simulink model "HANcoder_E407_GTSync_v6"  (R2018b)
settings: Solver=FixedStepDiscrete  StartTime=0.0  StopTime=1  FixedStep=0.01  RelTol=1e-3
PreLoadFcn:
  | librarySetup
  | eval([bdroot,'_startup']) %Calling [modelName]_startup.m
values from neighbouring files (symbols this model uses):
  basic_cycle_duration = TM_Reset_Board + COMP_duration    (= 212)    [HANcoder_E407_GTSync_v6_startup.m]
  comm_delay_estimation1 = round(comm_delay_measured1*hardware_granularity/frequency_IRQ)    [HANcoder_E407_GTSync_v6_startup.m]
  comm_delay_estimation2 = round(comm_delay_measured2*hardware_granularity/frequency_IRQ)    [HANcoder_E407_GTSync_v6_startup.m]
  COMM_Period = 40    [HANcoder_E407_GTSync_v6_startup.m]
  COMM_Phase1 = 5    [HANcoder_E407_GTSync_v6_startup.m]
  COMM_Phase2 = 8    [HANcoder_E407_GTSync_v6_startup.m]
  frequency_IRQ = 100    [HANcoder_E407_GTSync_v6_startup.m]
  HANtuneOverride = Simulink.Parameter    [HANcoder_E407_GTSync_v6_startup.m]
  idle_time_init = basic_cycle_duration*matrix_rows    (= 424)    [HANcoder_E407_GTSync_v6_startup.m]
  LA_COMM_Err = 1    [HANcoder_E407_GTSync_v6_startup.m]
  LA_MEX_Flag = 0    [HANcoder_E407_GTSync_v6_startup.m]
  LA_Task_Act = 1    [HANcoder_E407_GTSync_v6_startup.m]
  LED_ticks_toggle = 10000    [HANcoder_E407_GTSync_v6_startup.m]
  Master_Role = 1    [HANcoder_E407_GTSync_v6_startup.m]
  matrix_rows = 2    [HANcoder_E407_GTSync_v6_startup.m]
  max_num_msgs_CAN1 = 2^Tx_bit_number-1    (= 7)    [HANcoder_E407_GTSync_v6_startup.m]
  max_num_msgs_CAN2 = max_num_msgs_CAN1    (= 7)    [HANcoder_E407_GTSync_v6_startup.m]
  Slave_Role = 2    [HANcoder_E407_GTSync_v6_startup.m]
  Sync_ID = 1    [HANcoder_E407_GTSync_v6_startup.m]
  TM_Check_Sync = TM_COMM_Sync   + COMM_duration    (= 40)    [HANcoder_E407_GTSync_v6_startup.m]
  TM_Check_TOuts = TM_Count_Vote3 + COMP_duration    (= 196)    [HANcoder_E407_GTSync_v6_startup.m]
  TM_Check_Vote1 = TM_COMM_Vote1  + COMM_duration    (= 92)    [HANcoder_E407_GTSync_v6_startup.m]
  TM_Check_Vote2 = TM_COMM_Vote2  + COMM_duration    (= 140)    [HANcoder_E407_GTSync_v6_startup.m]
  TM_Check_Vote3 = TM_COMM_Vote3  + COMM_duration    (= 188)    [HANcoder_E407_GTSync_v6_startup.m]
  TM_COMM_Sync = basic_cycle_start    (= 0)    [HANcoder_E407_GTSync_v6_startup.m]
  TM_COMM_Vote1 = TM_Vote_Dec    + COMP_duration    (= 52)    [HANcoder_E407_GTSync_v6_startup.m]
  TM_COMM_Vote2 = TM_Count_Vote1 + COMP_duration    (= 100)    [HANcoder_E407_GTSync_v6_startup.m]
  TM_COMM_Vote3 = TM_Count_Vote2 + COMP_duration    (= 148)    [HANcoder_E407_GTSync_v6_startup.m]
  TM_Count_Vote1 = TM_Check_Vote1 + COMP_duration    (= 96)    [HANcoder_E407_GTSync_v6_startup.m]
  TM_Count_Vote2 = TM_Check_Vote2 + COMP_duration    (= 144)    [HANcoder_E407_GTSync_v6_startup.m]
  TM_Count_Vote3 = TM_Check_Vote3 + COMP_duration    (= 192)    [HANcoder_E407_GTSync_v6_startup.m]
  TM_Data = TM_COMM_Sync    (= 0)    [HANcoder_E407_GTSync_v6_startup.m]
  TM_New_Master = TM_Check_TOuts + COMP_duration    (= 200)    [HANcoder_E407_GTSync_v6_startup.m]
  TM_Reset_Board = TM_Reset_Var   + COMP_duration    (= 208)    [HANcoder_E407_GTSync_v6_startup.m]
  TM_Reset_Var = TM_New_Master  + COMP_duration    (= 204)    [HANcoder_E407_GTSync_v6_startup.m]
  TM_Type = COMM    (= 0)    [HANcoder_E407_GTSync_v6_startup.m]
  TM_Update_LT = TM_Check_Sync  + COMP_duration    (= 44)    [HANcoder_E407_GTSync_v6_startup.m]
  TM_Vote_Dec = TM_Update_LT   + COMP_duration    (= 48)    [HANcoder_E407_GTSync_v6_startup.m]
  Vote1_ID = 11    [HANcoder_E407_GTSync_v6_startup.m]
  Vote2_ID = 12    [HANcoder_E407_GTSync_v6_startup.m]
  Vote3_ID = 13    [HANcoder_E407_GTSync_v6_startup.m]
undefined symbols (not defined in the file or in its folder): A0, A1, A2, A3, CON2
libraries: hdlsllib x75, HANcoder_STM32_Target x25, simulink x3, simulink_extras x1
(part 3 of 8)

== system HANcoder_E407_GTSync_v6/HANcoder STM32 Target - E407-STM32 algorithm/Global Ticks Increment/CAN Management/Initialization/RoleID and Global Time init ==
  note: Sync msg received!
  note: Reset variables
  note: Finish Initialization
  note: Role_ID Initialization
  Timeout Initialization : Inport
  Reference message received : Inport  Port=2
  Enable : EnablePort
  Constant : Constant  Priority=4  Value=Master_Role
  Constant1 : Constant  Priority=3  Value=Slave_Role
  Data Store Read : DataStoreRead  Priority=5  DataStoreName=Role_ID
  Data Store Write : DataStoreWrite  Priority=8  DataStoreName=Role_ID
  Data Store Write2 : DataStoreWrite  Priority=18  DataStoreName=Delay_Counter
  Data Store Write3 : DataStoreWrite  Priority=12  DataStoreName=New_Msg_Ready_CAN1
  Data Store Write4 : DataStoreWrite  Priority=16  DataStoreName=Initialization_Timeout
  Data Store Write5 : DataStoreWrite  Priority=14  DataStoreName=New_Msg_Ready_CAN2
  Global Time Initialization Master : Subsystem  Priority=2
  Global Time Initialization Slave : Subsystem  Priority=1
  RESET : Constant  Priority=15  Value=0  OutDataTypeStr=boolean
  RESET1 : Constant  Priority=17  Value=0  OutDataTypeStr=double
  RESET2 : Constant  Priority=11  Value=0  OutDataTypeStr=boolean
  RESET3 : Constant  Priority=13  Value=0  OutDataTypeStr=boolean
  SET : Constant  Priority=19
  Switch1 : Switch  Priority=6  Criteria=u2 > Threshold
  Switch2 : Switch  Priority=7  Criteria=u2 > Threshold
  Finish Initialization : Outport  OutputWhenDisabled=reset  InitialOutput=0
  wires:
  Switch1/1 -> Switch2/3
  Reference message received/1 -> Global Time Initialization Slave/Enable, Switch2/2
  Data Store Read/1 -> Switch1/3
  SET/1 -> Finish Initialization/1
  Constant/1 -> Switch1/1
  Constant1/1 -> Switch2/1
  Switch2/1 -> Data Store Write/1
  RESET/1 -> Data Store Write4/1
  Timeout Initialization/1 -> Switch1/2, Global Time Initialization Master/Enable
  RESET1/1 -> Data Store Write2/1
  RESET2/1 -> Data Store Write3/1
  RESET3/1 -> Data Store Write5/1

== system HANcoder_E407_GTSync_v6/HANcoder STM32 Target - E407-STM32 algorithm/Global Ticks Increment/CAN Management/LT_Update Desync_Positive/Local Time Update with Positive Desync ==
  note: Positive Desync with respect to the master
      | If the desync is positive, we have to update the
      | Local Time to be "in the future". This is problematic
      | because we do not want the schedule to go ahead
      | of time and forget to do any task. That is why we
      | correct the desync in small steps.
  note: End condition
  note: Desync counter
      | reduction
  note: Local Time Update
  note: Current Local Time correction
  Ticks until next COMP : Inport
  Cast : DataTypeConversion  Priority=13  OutDataTypeStr=uint16
  Constant : Constant  Value=0
  Data Store Read : DataStoreRead  DataStoreName=Local_Ticks
  Data Store Read2 : DataStoreRead  DataStoreName=Desync_Ticks
  Data Store Write : DataStoreWrite  DataStoreName=Desync_Positive
  Data Store Write1 : DataStoreWrite  Priority=14  DataStoreName=Local_Ticks  DataStoreElements=Local_Ticks
  Data Store Write2 : DataStoreWrite  DataStoreName=Desync_Ticks
  Equal : RelationalOperator  Operator=<=  OutDataTypeStr=boolean  RndMeth=Simplest
  GreaterThan : RelationalOperator  Operator=<=  OutDataTypeStr=boolean  RndMeth=Simplest
  Minus : Sum  Priority=12
  Minus1 : Sum  Inputs=+-
  NOT : Logic  Operator=NOT  IconShape=distinctive  AllPortsSameDT=off  OutDataTypeStr=boolean
  Switch : Switch  Criteria=u2 > Threshold
  wires:
  Ticks until next COMP/1 -> Switch/1, GreaterThan/1
  Data Store Read/1 -> Minus/1
  Cast/1 -> Data Store Write1/1
  Minus/1 -> Cast/1
  Data Store Read2/1 -> Switch/3, GreaterThan/2, Minus1/2
  Minus1/1 -> Equal/1, Data Store Write2/1
  Constant/1 -> Equal/2
  Equal/1 -> NOT/1
  NOT/1 -> Data Store Write/1
  GreaterThan/1 -> Switch/2
  Switch/1 -> Minus1/1, Minus/2

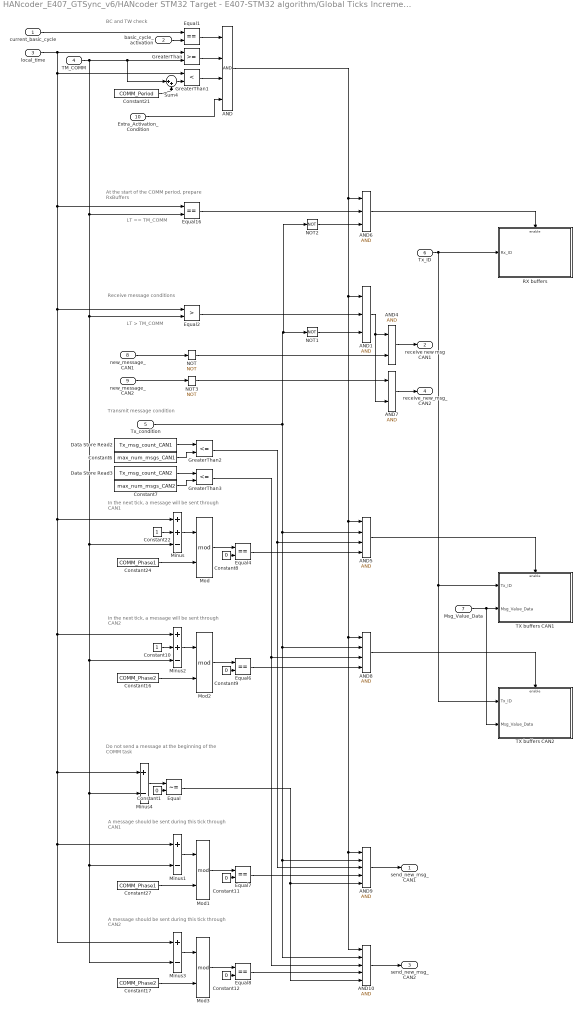
== system HANcoder_E407_GTSync_v6/HANcoder STM32 Target - E407-STM32 algorithm/Global Ticks Increment/CAN Management/Matrix Cycle Manager/COMM Task - Sync BC0 ==
  note: Do not send a message at the
      | beginning of the COMM task
  note: LT > TM_COMM
  note: At the start of the COMM
      | period, prepare RxBuffers
  note: In the next tick, a message will be
      | sent through CAN1
  note: BC and TW check
  note: Receive message conditions
  note: A message should be sent during
      | this tick through CAN1
  note: In the next tick, a message will be
      | sent through CAN2
  note: Transmit message condition
  note: A message should be sent during
      | this tick through CAN2
  note: LT == TM_COMM
  current_basic_cycle : Inport
  basic_cycle_activation : Inport  Port=2
  local_time : Inport  Port=3
  TM_COMM : Inport  Port=4
  Tx_condition : Inport  Port=5
  Tx_ID : Inport  Port=6
  Msg_Value_Data : Inport  Port=7
  new_message_CAN1 : Inport  Port=8
  new_message_CAN2 : Inport  Port=9
  Extra_Activation_Condition : Inport  Port=10
  AND : Logic  Inputs=4  IconShape=distinctive  AllPortsSameDT=off  OutDataTypeStr=boolean
  AND1 : Logic  Inputs=3  IconShape=distinctive  AllPortsSameDT=off  OutDataTypeStr=boolean
  AND10 : Logic  Inputs=5  IconShape=distinctive  AllPortsSameDT=off  OutDataTypeStr=boolean
  AND4 : Logic  IconShape=distinctive  AllPortsSameDT=off  OutDataTypeStr=boolean
  AND5 : Logic  Inputs=4  IconShape=distinctive  AllPortsSameDT=off  OutDataTypeStr=boolean
  AND6 : Logic  Inputs=3  IconShape=distinctive  AllPortsSameDT=off  OutDataTypeStr=boolean
  AND7 : Logic  IconShape=distinctive  AllPortsSameDT=off  OutDataTypeStr=boolean
  AND8 : Logic  Inputs=4  IconShape=distinctive  AllPortsSameDT=off  OutDataTypeStr=boolean
  AND9 : Logic  Inputs=5  IconShape=distinctive  AllPortsSameDT=off  OutDataTypeStr=boolean
  Constant{1,8..9,11..12} (5 alike) : Constant  Value=0
  Constant10 : Constant
  Constant16 : Constant  Value=COMM_Phase2
  Constant17 : Constant  Value=COMM_Phase2
  Constant21 : Constant  Value=COMM_Period
  Constant22 : Constant
  Constant24 : Constant  Value=COMM_Phase1
  Constant27 : Constant  Value=COMM_Phase1
  Constant6 : Constant  Value=max_num_msgs_CAN1
  Constant7 : Constant  Value=max_num_msgs_CAN2
  Data Store Read2 : DataStoreRead  DataStoreName=Tx_msg_count_CAN1
  Data Store Read3 : DataStoreRead  DataStoreName=Tx_msg_count_CAN2
  Equal : RelationalOperator  Operator=~=  OutDataTypeStr=boolean  RndMeth=Simplest
  Equal{1,4,6..8,16} (6 alike) : RelationalOperator  Operator===  OutDataTypeStr=boolean  RndMeth=Simplest
  Equal2 : RelationalOperator  Operator=>  OutDataTypeStr=boolean  RndMeth=Simplest
  GreaterThan : RelationalOperator  OutDataTypeStr=boolean  RndMeth=Simplest
  GreaterThan1 : RelationalOperator  Operator=<  OutDataTypeStr=boolean  RndMeth=Simplest
  GreaterThan2 : RelationalOperator  Operator=<=  OutDataTypeStr=boolean  RndMeth=Simplest
  GreaterThan3 : RelationalOperator  Operator=<=  OutDataTypeStr=boolean  RndMeth=Simplest
  Minus : Sum  Inputs=++-
  Minus1 : Sum  Inputs=+-
  Minus2 : Sum  Inputs=++-
  Minus3 : Sum  Inputs=+-
  Minus4 : Sum  Inputs=+-
  Mod{,1..3} (4 alike) : Math  Operator=mod  SaturateOnIntegerOverflow=on
  NOT{,1..3} (4 alike) : Logic  Operator=NOT  IconShape=distinctive  AllPortsSameDT=off  OutDataTypeStr=boolean
  RX buffers : Subsystem  Priority=20
  Sum4 : Sum  Inputs=|++
  TX buffers CAN1 : Subsystem  Priority=20
  TX buffers CAN2 : Subsystem  Priority=20
  send_new_msg_CAN1 : Outport
  receive new msg CAN1 : Outport  Port=2
  send_new_msg_CAN2 : Outport  Port=3
  receive_new_msg_CAN2 : Outport  Port=4
  wires:
  basic_cycle_activation/1 -> Equal1/2
  new_message_CAN1/1 -> NOT/1
  current_basic_cycle/1 -> Equal1/1
  Constant21/1 -> Sum4/2
  Sum4/1 -> GreaterThan1/2
  Equal1/1 -> AND/1
  GreaterThan/1 -> AND/2
  GreaterThan1/1 -> AND/3
  AND5/1 -> TX buffers CAN1/Enable
  Constant22/1 -> Minus/2
  Minus/1 -> Mod/1
  Constant24/1 -> Mod/2
  Constant27/1 -> Mod1/2
  Minus1/1 -> Mod1/1
  Equal16/1 -> AND6/2
  AND6/1 -> RX buffers/Enable
  NOT3/1 -> AND7/1
  new_message_CAN2/1 -> NOT3/1
  Equal2/1 -> AND1/2
  Tx_condition/1 -> NOT2/1, NOT1/1, AND10/2, AND9/2, AND8/2, AND5/2
  AND1/1 -> AND4/1, AND7/2
  NOT/1 -> AND4/2
  AND4/1 -> receive new msg CAN1/1
  AND7/1 -> receive_new_msg_CAN2/1
  Constant16/1 -> Mod2/2
  Minus2/1 -> Mod2/1
  Constant10/1 -> Minus2/2
  AND8/1 -> TX buffers CAN2/Enable
  AND9/1 -> send_new_msg_CAN1/1
  AND10/1 -> send_new_msg_CAN2/1
  AND/1 -> AND8/1, AND9/1, AND10/1, AND5/1, AND1/1, AND6/1
  TM_COMM/1 -> Minus/3, Minus2/3, Minus4/2, Minus3/2, Minus1/2, Equal2/2, Equal16/2, Sum4/1, GreaterThan/2
  Minus3/1 -> Mod3/1
  Constant17/1 -> Mod3/2
  Data Store Read2/1 -> GreaterThan2/1
  Constant6/1 -> GreaterThan2/2
  Constant7/1 -> GreaterThan3/2
  Data Store Read3/1 -> GreaterThan3/1
  GreaterThan2/1 -> AND9/3, AND5/3
  GreaterThan3/1 -> AND10/3, AND8/3
  Equal4/1 -> AND5/4
  Mod/1 -> Equal4/1
  Constant8/1 -> Equal4/2
  Constant9/1 -> Equal6/2
  Mod2/1 -> Equal6/1
  Constant11/1 -> Equal7/2
  Constant12/1 -> Equal8/2
  Mod3/1 -> Equal8/1
  Mod1/1 -> Equal7/1
  Equal6/1 -> AND8/4
  Equal7/1 -> AND9/4
  Equal8/1 -> AND10/4
  Tx_ID/1 -> RX buffers/1(Rx_ID), TX buffers CAN1/1(Tx_ID), TX buffers CAN2/1(Tx_ID)
  NOT1/1 -> AND1/3
  Extra_Activation_Condition/1 -> AND/4
  Msg_Value_Data/1 -> TX buffers CAN2/2(Msg_Value_Data), TX buffers CAN1/2(Msg_Value_Data)
  local_time/1 -> GreaterThan1/1, Equal16/1, Equal2/1, Minus3/1, Minus1/1, Minus4/1, Minus2/1, Minus/1, GreaterThan/1
  NOT2/1 -> AND6/3
  Constant1/1 -> Equal/2
  Minus4/1 -> Equal/1
  Equal/1 -> AND10/5, AND9/5

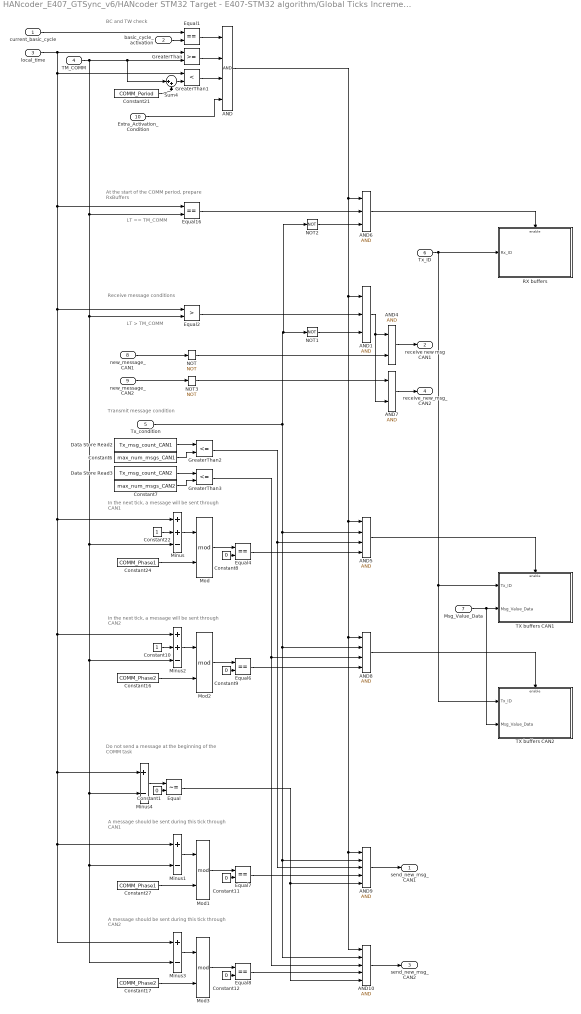
== system HANcoder_E407_GTSync_v6/HANcoder STM32 Target - E407-STM32 algorithm/Global Ticks Increment/CAN Management/Matrix Cycle Manager/COMM Task - Sync BC1 ==
  note: Do not send a message at the
      | beginning of the COMM task
  note: LT > TM_COMM
  note: At the start of the COMM
      | period, prepare RxBuffers
  note: In the next tick, a message will be
      | sent through CAN1
  note: BC and TW check
  note: Receive message conditions
  note: A message should be sent during
      | this tick through CAN1
  note: In the next tick, a message will be
      | sent through CAN2
  note: Transmit message condition
  note: A message should be sent during
      | this tick through CAN2
  note: LT == TM_COMM
  current_basic_cycle : Inport
  basic_cycle_activation : Inport  Port=2
  local_time : Inport  Port=3
  TM_COMM : Inport  Port=4
  Tx_condition : Inport  Port=5
  Tx_ID : Inport  Port=6
  Msg_Value_Data : Inport  Port=7
  new_message_CAN1 : Inport  Port=8
  new_message_CAN2 : Inport  Port=9
  Extra_Activation_Condition : Inport  Port=10
  AND : Logic  Inputs=4  IconShape=distinctive  AllPortsSameDT=off  OutDataTypeStr=boolean
  AND1 : Logic  Inputs=3  IconShape=distinctive  AllPortsSameDT=off  OutDataTypeStr=boolean
  AND10 : Logic  Inputs=5  IconShape=distinctive  AllPortsSameDT=off  OutDataTypeStr=boolean
  AND4 : Logic  IconShape=distinctive  AllPortsSameDT=off  OutDataTypeStr=boolean
  AND5 : Logic  Inputs=4  IconShape=distinctive  AllPortsSameDT=off  OutDataTypeStr=boolean
  AND6 : Logic  Inputs=3  IconShape=distinctive  AllPortsSameDT=off  OutDataTypeStr=boolean
  AND7 : Logic  IconShape=distinctive  AllPortsSameDT=off  OutDataTypeStr=boolean
  AND8 : Logic  Inputs=4  IconShape=distinctive  AllPortsSameDT=off  OutDataTypeStr=boolean
  AND9 : Logic  Inputs=5  IconShape=distinctive  AllPortsSameDT=off  OutDataTypeStr=boolean
  Constant{1,8..9,11..12} (5 alike) : Constant  Value=0
  Constant10 : Constant
  Constant16 : Constant  Value=COMM_Phase2
  Constant17 : Constant  Value=COMM_Phase2
  Constant21 : Constant  Value=COMM_Period
  Constant22 : Constant
  Constant24 : Constant  Value=COMM_Phase1
  Constant27 : Constant  Value=COMM_Phase1
  Constant6 : Constant  Value=max_num_msgs_CAN1
  Constant7 : Constant  Value=max_num_msgs_CAN2
  Data Store Read2 : DataStoreRead  DataStoreName=Tx_msg_count_CAN1
  Data Store Read3 : DataStoreRead  DataStoreName=Tx_msg_count_CAN2
  Equal : RelationalOperator  Operator=~=  OutDataTypeStr=boolean  RndMeth=Simplest
  Equal{1,4,6..8,16} (6 alike) : RelationalOperator  Operator===  OutDataTypeStr=boolean  RndMeth=Simplest
  Equal2 : RelationalOperator  Operator=>  OutDataTypeStr=boolean  RndMeth=Simplest
  GreaterThan : RelationalOperator  OutDataTypeStr=boolean  RndMeth=Simplest
  GreaterThan1 : RelationalOperator  Operator=<  OutDataTypeStr=boolean  RndMeth=Simplest
  GreaterThan2 : RelationalOperator  Operator=<=  OutDataTypeStr=boolean  RndMeth=Simplest
  GreaterThan3 : RelationalOperator  Operator=<=  OutDataTypeStr=boolean  RndMeth=Simplest
  Minus : Sum  Inputs=++-
  Minus1 : Sum  Inputs=+-
  Minus2 : Sum  Inputs=++-
  Minus3 : Sum  Inputs=+-
  Minus4 : Sum  Inputs=+-
  Mod{,1..3} (4 alike) : Math  Operator=mod  SaturateOnIntegerOverflow=on
  NOT{,1..3} (4 alike) : Logic  Operator=NOT  IconShape=distinctive  AllPortsSameDT=off  OutDataTypeStr=boolean
  RX buffers : Subsystem  Priority=20
  Sum4 : Sum  Inputs=|++
  TX buffers CAN1 : Subsystem  Priority=20
  TX buffers CAN2 : Subsystem  Priority=20
  send_new_msg_CAN1 : Outport
  receive new msg CAN1 : Outport  Port=2
  send_new_msg_CAN2 : Outport  Port=3
  receive_new_msg_CAN2 : Outport  Port=4
  wires:
  basic_cycle_activation/1 -> Equal1/2
  new_message_CAN1/1 -> NOT/1
  current_basic_cycle/1 -> Equal1/1
  Constant21/1 -> Sum4/2
  Sum4/1 -> GreaterThan1/2
  Equal1/1 -> AND/1
  GreaterThan/1 -> AND/2
  GreaterThan1/1 -> AND/3
  AND5/1 -> TX buffers CAN1/Enable
  Constant22/1 -> Minus/2
  Minus/1 -> Mod/1
  Constant24/1 -> Mod/2
  Constant27/1 -> Mod1/2
  Minus1/1 -> Mod1/1
  Equal16/1 -> AND6/2
  AND6/1 -> RX buffers/Enable
  NOT3/1 -> AND7/1
  new_message_CAN2/1 -> NOT3/1
  Equal2/1 -> AND1/2
  Tx_condition/1 -> NOT2/1, NOT1/1, AND10/2, AND9/2, AND8/2, AND5/2
  AND1/1 -> AND4/1, AND7/2
  NOT/1 -> AND4/2
  AND4/1 -> receive new msg CAN1/1
  AND7/1 -> receive_new_msg_CAN2/1
  Constant16/1 -> Mod2/2
  Minus2/1 -> Mod2/1
  Constant10/1 -> Minus2/2
  AND8/1 -> TX buffers CAN2/Enable
  AND9/1 -> send_new_msg_CAN1/1
  AND10/1 -> send_new_msg_CAN2/1
  AND/1 -> AND8/1, AND9/1, AND10/1, AND5/1, AND1/1, AND6/1
  TM_COMM/1 -> Minus/3, Minus2/3, Minus4/2, Minus3/2, Minus1/2, Equal2/2, Equal16/2, Sum4/1, GreaterThan/2
  Minus3/1 -> Mod3/1
  Constant17/1 -> Mod3/2
  Data Store Read2/1 -> GreaterThan2/1
  Constant6/1 -> GreaterThan2/2
  Constant7/1 -> GreaterThan3/2
  Data Store Read3/1 -> GreaterThan3/1
  GreaterThan2/1 -> AND9/3, AND5/3
  GreaterThan3/1 -> AND10/3, AND8/3
  Equal4/1 -> AND5/4
  Mod/1 -> Equal4/1
  Constant8/1 -> Equal4/2
  Constant9/1 -> Equal6/2
  Mod2/1 -> Equal6/1
  Constant11/1 -> Equal7/2
  Constant12/1 -> Equal8/2
  Mod3/1 -> Equal8/1
  Mod1/1 -> Equal7/1
  Equal6/1 -> AND8/4
  Equal7/1 -> AND9/4
  Equal8/1 -> AND10/4
  Tx_ID/1 -> RX buffers/1(Rx_ID), TX buffers CAN1/1(Tx_ID), TX buffers CAN2/1(Tx_ID)
  NOT1/1 -> AND1/3
  Extra_Activation_Condition/1 -> AND/4
  Msg_Value_Data/1 -> TX buffers CAN2/2(Msg_Value_Data), TX buffers CAN1/2(Msg_Value_Data)
  local_time/1 -> GreaterThan1/1, Equal16/1, Equal2/1, Minus3/1, Minus1/1, Minus4/1, Minus2/1, Minus/1, GreaterThan/1
  NOT2/1 -> AND6/3
  Constant1/1 -> Equal/2
  Minus4/1 -> Equal/1
  Equal/1 -> AND10/5, AND9/5

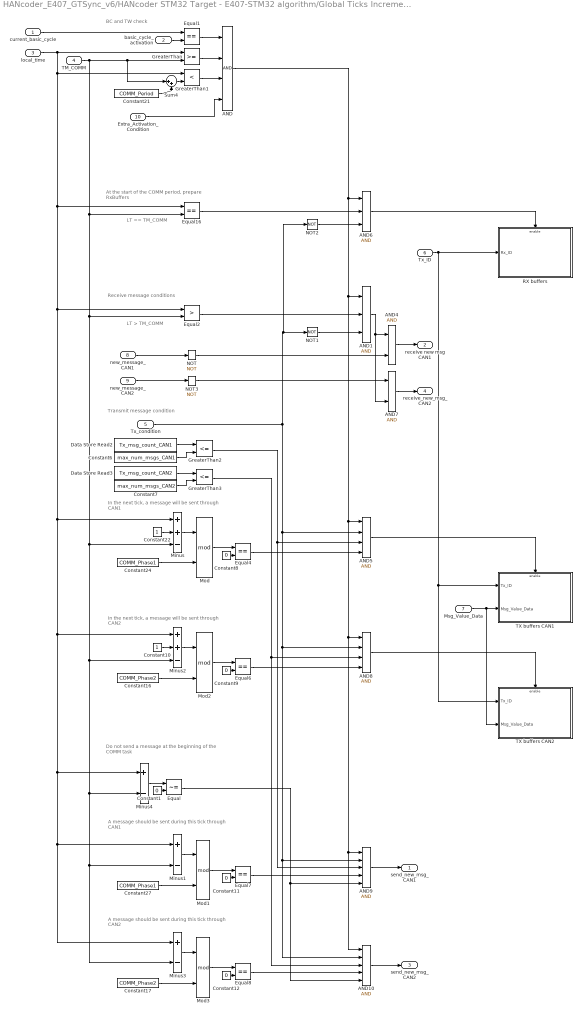
== system HANcoder_E407_GTSync_v6/HANcoder STM32 Target - E407-STM32 algorithm/Global Ticks Increment/CAN Management/Matrix Cycle Manager/COMM Task - Vote1 ==
  note: Do not send a message at the
      | beginning of the COMM task
  note: LT > TM_COMM
  note: At the start of the COMM
      | period, prepare RxBuffers
  note: In the next tick, a message will be
      | sent through CAN1
  note: BC and TW check
  note: Receive message conditions
  note: A message should be sent during
      | this tick through CAN1
  note: In the next tick, a message will be
      | sent through CAN2
  note: Transmit message condition
  note: A message should be sent during
      | this tick through CAN2
  note: LT == TM_COMM
  current_basic_cycle : Inport
  basic_cycle_activation : Inport  Port=2
  local_time : Inport  Port=3
  TM_COMM : Inport  Port=4
  Tx_condition : Inport  Port=5
  Tx_ID : Inport  Port=6
  Msg_Value_Data : Inport  Port=7
  new_message_CAN1 : Inport  Port=8
  new_message_CAN2 : Inport  Port=9
  Extra_Activation_Condition : Inport  Port=10
  AND : Logic  Inputs=4  IconShape=distinctive  AllPortsSameDT=off  OutDataTypeStr=boolean
  AND1 : Logic  Inputs=3  IconShape=distinctive  AllPortsSameDT=off  OutDataTypeStr=boolean
  AND10 : Logic  Inputs=5  IconShape=distinctive  AllPortsSameDT=off  OutDataTypeStr=boolean
  AND4 : Logic  IconShape=distinctive  AllPortsSameDT=off  OutDataTypeStr=boolean
  AND5 : Logic  Inputs=4  IconShape=distinctive  AllPortsSameDT=off  OutDataTypeStr=boolean
  AND6 : Logic  Inputs=3  IconShape=distinctive  AllPortsSameDT=off  OutDataTypeStr=boolean
  AND7 : Logic  IconShape=distinctive  AllPortsSameDT=off  OutDataTypeStr=boolean
  AND8 : Logic  Inputs=4  IconShape=distinctive  AllPortsSameDT=off  OutDataTypeStr=boolean
  AND9 : Logic  Inputs=5  IconShape=distinctive  AllPortsSameDT=off  OutDataTypeStr=boolean
  Constant{1,8..9,11..12} (5 alike) : Constant  Value=0
  Constant10 : Constant
  Constant16 : Constant  Value=COMM_Phase2
  Constant17 : Constant  Value=COMM_Phase2
  Constant21 : Constant  Value=COMM_Period
  Constant22 : Constant
  Constant24 : Constant  Value=COMM_Phase1
  Constant27 : Constant  Value=COMM_Phase1
  Constant6 : Constant  Value=max_num_msgs_CAN1
  Constant7 : Constant  Value=max_num_msgs_CAN2
  Data Store Read2 : DataStoreRead  DataStoreName=Tx_msg_count_CAN1
  Data Store Read3 : DataStoreRead  DataStoreName=Tx_msg_count_CAN2
  Equal : RelationalOperator  Operator=~=  OutDataTypeStr=boolean  RndMeth=Simplest
  Equal{1,4,6..8,16} (6 alike) : RelationalOperator  Operator===  OutDataTypeStr=boolean  RndMeth=Simplest
  Equal2 : RelationalOperator  Operator=>  OutDataTypeStr=boolean  RndMeth=Simplest
  GreaterThan : RelationalOperator  OutDataTypeStr=boolean  RndMeth=Simplest
  GreaterThan1 : RelationalOperator  Operator=<  OutDataTypeStr=boolean  RndMeth=Simplest
  GreaterThan2 : RelationalOperator  Operator=<=  OutDataTypeStr=boolean  RndMeth=Simplest
  GreaterThan3 : RelationalOperator  Operator=<=  OutDataTypeStr=boolean  RndMeth=Simplest
  Minus : Sum  Inputs=++-
  Minus1 : Sum  Inputs=+-
  Minus2 : Sum  Inputs=++-
  Minus3 : Sum  Inputs=+-
  Minus4 : Sum  Inputs=+-
  Mod{,1..3} (4 alike) : Math  Operator=mod  SaturateOnIntegerOverflow=on
  NOT{,1..3} (4 alike) : Logic  Operator=NOT  IconShape=distinctive  AllPortsSameDT=off  OutDataTypeStr=boolean
  RX buffers : Subsystem  Priority=20
  Sum4 : Sum  Inputs=|++
  TX buffers CAN1 : Subsystem  Priority=20
  TX buffers CAN2 : Subsystem  Priority=20
  send_new_msg_CAN1 : Outport
  receive new msg CAN1 : Outport  Port=2
  send_new_msg_CAN2 : Outport  Port=3
  receive_new_msg_CAN2 : Outport  Port=4
  wires:
  basic_cycle_activation/1 -> Equal1/2
  new_message_CAN1/1 -> NOT/1
  current_basic_cycle/1 -> Equal1/1
  Constant21/1 -> Sum4/2
  Sum4/1 -> GreaterThan1/2
  Equal1/1 -> AND/1
  GreaterThan/1 -> AND/2
  GreaterThan1/1 -> AND/3
  AND5/1 -> TX buffers CAN1/Enable
  Constant22/1 -> Minus/2
  Minus/1 -> Mod/1
  Constant24/1 -> Mod/2
  Constant27/1 -> Mod1/2
  Minus1/1 -> Mod1/1
  Equal16/1 -> AND6/2
  AND6/1 -> RX buffers/Enable
  NOT3/1 -> AND7/1
  new_message_CAN2/1 -> NOT3/1
  Equal2/1 -> AND1/2
  Tx_condition/1 -> NOT2/1, NOT1/1, AND10/2, AND9/2, AND8/2, AND5/2
  AND1/1 -> AND4/1, AND7/2
  NOT/1 -> AND4/2
  AND4/1 -> receive new msg CAN1/1
  AND7/1 -> receive_new_msg_CAN2/1
  Constant16/1 -> Mod2/2
  Minus2/1 -> Mod2/1
  Constant10/1 -> Minus2/2
  AND8/1 -> TX buffers CAN2/Enable
  AND9/1 -> send_new_msg_CAN1/1
  AND10/1 -> send_new_msg_CAN2/1
  AND/1 -> AND8/1, AND9/1, AND10/1, AND5/1, AND1/1, AND6/1
  TM_COMM/1 -> Minus/3, Minus2/3, Minus4/2, Minus3/2, Minus1/2, Equal2/2, Equal16/2, Sum4/1, GreaterThan/2
  Minus3/1 -> Mod3/1
  Constant17/1 -> Mod3/2
  Data Store Read2/1 -> GreaterThan2/1
  Constant6/1 -> GreaterThan2/2
  Constant7/1 -> GreaterThan3/2
  Data Store Read3/1 -> GreaterThan3/1
  GreaterThan2/1 -> AND9/3, AND5/3
  GreaterThan3/1 -> AND10/3, AND8/3
  Equal4/1 -> AND5/4
  Mod/1 -> Equal4/1
  Constant8/1 -> Equal4/2
  Constant9/1 -> Equal6/2
  Mod2/1 -> Equal6/1
  Constant11/1 -> Equal7/2
  Constant12/1 -> Equal8/2
  Mod3/1 -> Equal8/1
  Mod1/1 -> Equal7/1
  Equal6/1 -> AND8/4
  Equal7/1 -> AND9/4
  Equal8/1 -> AND10/4
  Tx_ID/1 -> RX buffers/1(Rx_ID), TX buffers CAN1/1(Tx_ID), TX buffers CAN2/1(Tx_ID)
  NOT1/1 -> AND1/3
  Extra_Activation_Condition/1 -> AND/4
  Msg_Value_Data/1 -> TX buffers CAN2/2(Msg_Value_Data), TX buffers CAN1/2(Msg_Value_Data)
  local_time/1 -> GreaterThan1/1, Equal16/1, Equal2/1, Minus3/1, Minus1/1, Minus4/1, Minus2/1, Minus/1, GreaterThan/1
  NOT2/1 -> AND6/3
  Constant1/1 -> Equal/2
  Minus4/1 -> Equal/1
  Equal/1 -> AND10/5, AND9/5

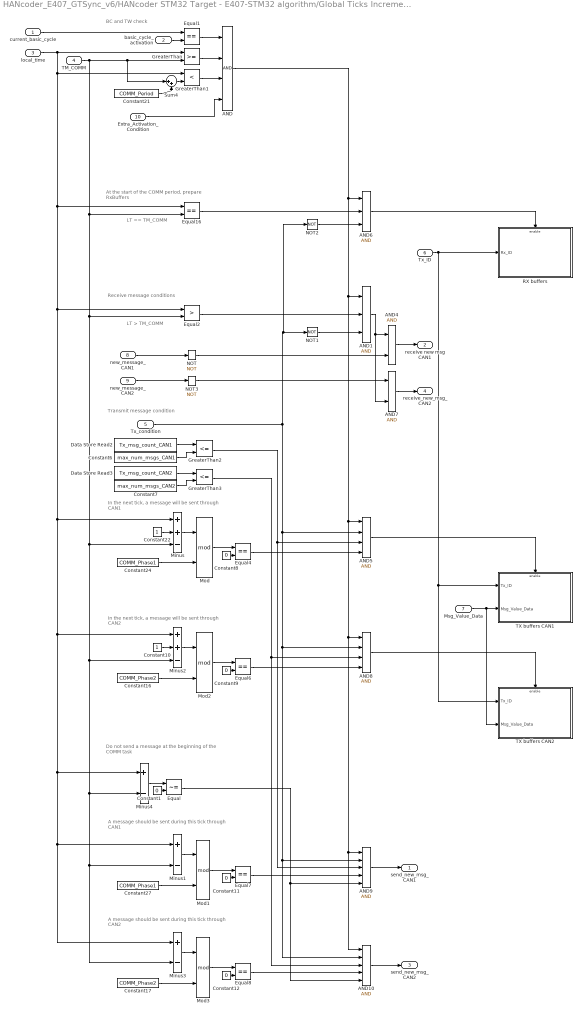
== system HANcoder_E407_GTSync_v6/HANcoder STM32 Target - E407-STM32 algorithm/Global Ticks Increment/CAN Management/Matrix Cycle Manager/COMM Task - Vote2 ==
  note: Do not send a message at the
      | beginning of the COMM task
  note: LT > TM_COMM
  note: At the start of the COMM
      | period, prepare RxBuffers
  note: In the next tick, a message will be
      | sent through CAN1
  note: BC and TW check
  note: Receive message conditions
  note: A message should be sent during
      | this tick through CAN1
  note: In the next tick, a message will be
      | sent through CAN2
  note: Transmit message condition
  note: A message should be sent during
      | this tick through CAN2
  note: LT == TM_COMM
  current_basic_cycle : Inport
  basic_cycle_activation : Inport  Port=2
  local_time : Inport  Port=3
  TM_COMM : Inport  Port=4
  Tx_condition : Inport  Port=5
  Tx_ID : Inport  Port=6
  Msg_Value_Data : Inport  Port=7
  new_message_CAN1 : Inport  Port=8
  new_message_CAN2 : Inport  Port=9
  Extra_Activation_Condition : Inport  Port=10
  AND : Logic  Inputs=4  IconShape=distinctive  AllPortsSameDT=off  OutDataTypeStr=boolean
  AND1 : Logic  Inputs=3  IconShape=distinctive  AllPortsSameDT=off  OutDataTypeStr=boolean
  AND10 : Logic  Inputs=5  IconShape=distinctive  AllPortsSameDT=off  OutDataTypeStr=boolean
  AND4 : Logic  IconShape=distinctive  AllPortsSameDT=off  OutDataTypeStr=boolean
  AND5 : Logic  Inputs=4  IconShape=distinctive  AllPortsSameDT=off  OutDataTypeStr=boolean
  AND6 : Logic  Inputs=3  IconShape=distinctive  AllPortsSameDT=off  OutDataTypeStr=boolean
  AND7 : Logic  IconShape=distinctive  AllPortsSameDT=off  OutDataTypeStr=boolean
  AND8 : Logic  Inputs=4  IconShape=distinctive  AllPortsSameDT=off  OutDataTypeStr=boolean
  AND9 : Logic  Inputs=5  IconShape=distinctive  AllPortsSameDT=off  OutDataTypeStr=boolean
  Constant{1,8..9,11..12} (5 alike) : Constant  Value=0
  Constant10 : Constant
  Constant16 : Constant  Value=COMM_Phase2
  Constant17 : Constant  Value=COMM_Phase2
  Constant21 : Constant  Value=COMM_Period
  Constant22 : Constant
  Constant24 : Constant  Value=COMM_Phase1
  Constant27 : Constant  Value=COMM_Phase1
  Constant6 : Constant  Value=max_num_msgs_CAN1
  Constant7 : Constant  Value=max_num_msgs_CAN2
  Data Store Read2 : DataStoreRead  DataStoreName=Tx_msg_count_CAN1
  Data Store Read3 : DataStoreRead  DataStoreName=Tx_msg_count_CAN2
  Equal : RelationalOperator  Operator=~=  OutDataTypeStr=boolean  RndMeth=Simplest
  Equal{1,4,6..8,16} (6 alike) : RelationalOperator  Operator===  OutDataTypeStr=boolean  RndMeth=Simplest
  Equal2 : RelationalOperator  Operator=>  OutDataTypeStr=boolean  RndMeth=Simplest
  GreaterThan : RelationalOperator  OutDataTypeStr=boolean  RndMeth=Simplest
  GreaterThan1 : RelationalOperator  Operator=<  OutDataTypeStr=boolean  RndMeth=Simplest
  GreaterThan2 : RelationalOperator  Operator=<=  OutDataTypeStr=boolean  RndMeth=Simplest
  GreaterThan3 : RelationalOperator  Operator=<=  OutDataTypeStr=boolean  RndMeth=Simplest
  Minus : Sum  Inputs=++-
  Minus1 : Sum  Inputs=+-
  Minus2 : Sum  Inputs=++-
  Minus3 : Sum  Inputs=+-
  Minus4 : Sum  Inputs=+-
  Mod{,1..3} (4 alike) : Math  Operator=mod  SaturateOnIntegerOverflow=on
  NOT{,1..3} (4 alike) : Logic  Operator=NOT  IconShape=distinctive  AllPortsSameDT=off  OutDataTypeStr=boolean
  RX buffers : Subsystem  Priority=20
  Sum4 : Sum  Inputs=|++
  TX buffers CAN1 : Subsystem  Priority=20
  TX buffers CAN2 : Subsystem  Priority=20
  send_new_msg_CAN1 : Outport
  receive new msg CAN1 : Outport  Port=2
  send_new_msg_CAN2 : Outport  Port=3
  receive_new_msg_CAN2 : Outport  Port=4
  wires:
  basic_cycle_activation/1 -> Equal1/2
  new_message_CAN1/1 -> NOT/1
  current_basic_cycle/1 -> Equal1/1
  Constant21/1 -> Sum4/2
  Sum4/1 -> GreaterThan1/2
  Equal1/1 -> AND/1
  GreaterThan/1 -> AND/2
  GreaterThan1/1 -> AND/3
  AND5/1 -> TX buffers CAN1/Enable
  Constant22/1 -> Minus/2
  Minus/1 -> Mod/1
  Constant24/1 -> Mod/2
  Constant27/1 -> Mod1/2
  Minus1/1 -> Mod1/1
  Equal16/1 -> AND6/2
  AND6/1 -> RX buffers/Enable
  NOT3/1 -> AND7/1
  new_message_CAN2/1 -> NOT3/1
  Equal2/1 -> AND1/2
  Tx_condition/1 -> NOT2/1, NOT1/1, AND10/2, AND9/2, AND8/2, AND5/2
  AND1/1 -> AND4/1, AND7/2
  NOT/1 -> AND4/2
  AND4/1 -> receive new msg CAN1/1
  AND7/1 -> receive_new_msg_CAN2/1
  Constant16/1 -> Mod2/2
  Minus2/1 -> Mod2/1
  Constant10/1 -> Minus2/2
  AND8/1 -> TX buffers CAN2/Enable
  AND9/1 -> send_new_msg_CAN1/1
  AND10/1 -> send_new_msg_CAN2/1
  AND/1 -> AND8/1, AND9/1, AND10/1, AND5/1, AND1/1, AND6/1
  TM_COMM/1 -> Minus/3, Minus2/3, Minus4/2, Minus3/2, Minus1/2, Equal2/2, Equal16/2, Sum4/1, GreaterThan/2
  Minus3/1 -> Mod3/1
  Constant17/1 -> Mod3/2
  Data Store Read2/1 -> GreaterThan2/1
  Constant6/1 -> GreaterThan2/2
  Constant7/1 -> GreaterThan3/2
  Data Store Read3/1 -> GreaterThan3/1
  GreaterThan2/1 -> AND9/3, AND5/3
  GreaterThan3/1 -> AND10/3, AND8/3
  Equal4/1 -> AND5/4
  Mod/1 -> Equal4/1
  Constant8/1 -> Equal4/2
  Constant9/1 -> Equal6/2
  Mod2/1 -> Equal6/1
  Constant11/1 -> Equal7/2
  Constant12/1 -> Equal8/2
  Mod3/1 -> Equal8/1
  Mod1/1 -> Equal7/1
  Equal6/1 -> AND8/4
  Equal7/1 -> AND9/4
  Equal8/1 -> AND10/4
  Tx_ID/1 -> RX buffers/1(Rx_ID), TX buffers CAN1/1(Tx_ID), TX buffers CAN2/1(Tx_ID)
  NOT1/1 -> AND1/3
  Extra_Activation_Condition/1 -> AND/4
  Msg_Value_Data/1 -> TX buffers CAN2/2(Msg_Value_Data), TX buffers CAN1/2(Msg_Value_Data)
  local_time/1 -> GreaterThan1/1, Equal16/1, Equal2/1, Minus3/1, Minus1/1, Minus4/1, Minus2/1, Minus/1, GreaterThan/1
  NOT2/1 -> AND6/3
  Constant1/1 -> Equal/2
  Minus4/1 -> Equal/1
  Equal/1 -> AND10/5, AND9/5

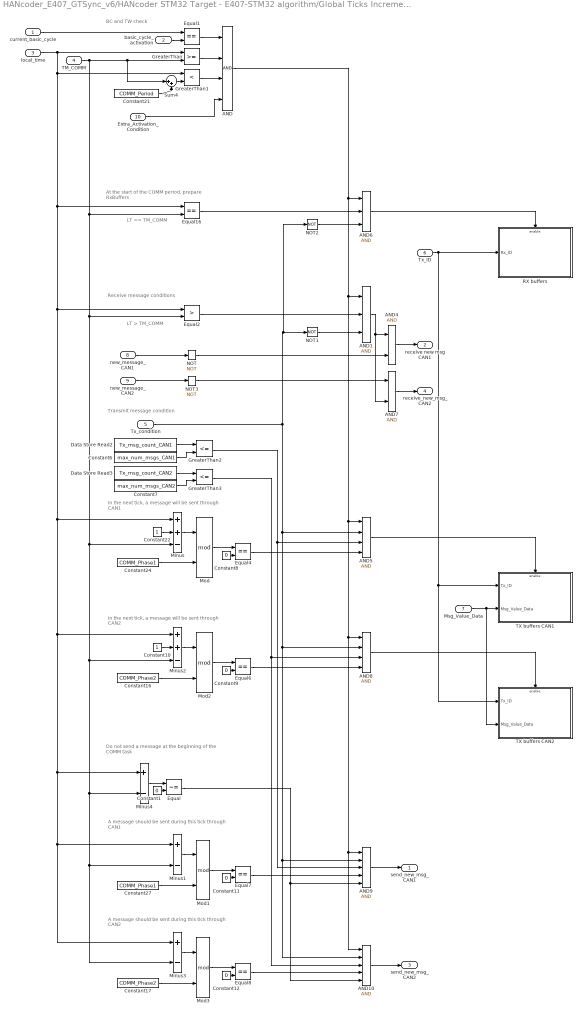
== system HANcoder_E407_GTSync_v6/HANcoder STM32 Target - E407-STM32 algorithm/Global Ticks Increment/CAN Management/Matrix Cycle Manager/COMM Task - Vote3 ==
  note: Do not send a message at the
      | beginning of the COMM task
  note: LT > TM_COMM
  note: At the start of the COMM
      | period, prepare RxBuffers
  note: In the next tick, a message will be
      | sent through CAN1
  note: BC and TW check
  note: Receive message conditions
  note: A message should be sent during
      | this tick through CAN1
  note: In the next tick, a message will be
      | sent through CAN2
  note: Transmit message condition
  note: A message should be sent during
      | this tick through CAN2
  note: LT == TM_COMM
  current_basic_cycle : Inport
  basic_cycle_activation : Inport  Port=2
  local_time : Inport  Port=3
  TM_COMM : Inport  Port=4
  Tx_condition : Inport  Port=5
  Tx_ID : Inport  Port=6
  Msg_Value_Data : Inport  Port=7
  new_message_CAN1 : Inport  Port=8
  new_message_CAN2 : Inport  Port=9
  Extra_Activation_Condition : Inport  Port=10
  AND : Logic  Inputs=4  IconShape=distinctive  AllPortsSameDT=off  OutDataTypeStr=boolean
  AND1 : Logic  Inputs=3  IconShape=distinctive  AllPortsSameDT=off  OutDataTypeStr=boolean
  AND10 : Logic  Inputs=5  IconShape=distinctive  AllPortsSameDT=off  OutDataTypeStr=boolean
  AND4 : Logic  IconShape=distinctive  AllPortsSameDT=off  OutDataTypeStr=boolean
  AND5 : Logic  Inputs=4  IconShape=distinctive  AllPortsSameDT=off  OutDataTypeStr=boolean
  AND6 : Logic  Inputs=3  IconShape=distinctive  AllPortsSameDT=off  OutDataTypeStr=boolean
  AND7 : Logic  IconShape=distinctive  AllPortsSameDT=off  OutDataTypeStr=boolean
  AND8 : Logic  Inputs=4  IconShape=distinctive  AllPortsSameDT=off  OutDataTypeStr=boolean
  AND9 : Logic  Inputs=5  IconShape=distinctive  AllPortsSameDT=off  OutDataTypeStr=boolean
  Constant{1,8..9,11..12} (5 alike) : Constant  Value=0
  Constant10 : Constant
  Constant16 : Constant  Value=COMM_Phase2
  Constant17 : Constant  Value=COMM_Phase2
  Constant21 : Constant  Value=COMM_Period
  Constant22 : Constant
  Constant24 : Constant  Value=COMM_Phase1
  Constant27 : Constant  Value=COMM_Phase1
  Constant6 : Constant  Value=max_num_msgs_CAN1
  Constant7 : Constant  Value=max_num_msgs_CAN2
  Data Store Read2 : DataStoreRead  DataStoreName=Tx_msg_count_CAN1
  Data Store Read3 : DataStoreRead  DataStoreName=Tx_msg_count_CAN2
  Equal : RelationalOperator  Operator=~=  OutDataTypeStr=boolean  RndMeth=Simplest
  Equal{1,4,6..8,16} (6 alike) : RelationalOperator  Operator===  OutDataTypeStr=boolean  RndMeth=Simplest
  Equal2 : RelationalOperator  Operator=>  OutDataTypeStr=boolean  RndMeth=Simplest
  GreaterThan : RelationalOperator  OutDataTypeStr=boolean  RndMeth=Simplest
  GreaterThan1 : RelationalOperator  Operator=<  OutDataTypeStr=boolean  RndMeth=Simplest
  GreaterThan2 : RelationalOperator  Operator=<=  OutDataTypeStr=boolean  RndMeth=Simplest
  GreaterThan3 : RelationalOperator  Operator=<=  OutDataTypeStr=boolean  RndMeth=Simplest
  Minus : Sum  Inputs=++-
  Minus1 : Sum  Inputs=+-
  Minus2 : Sum  Inputs=++-
  Minus3 : Sum  Inputs=+-
  Minus4 : Sum  Inputs=+-
  Mod{,1..3} (4 alike) : Math  Operator=mod  SaturateOnIntegerOverflow=on
  NOT{,1..3} (4 alike) : Logic  Operator=NOT  IconShape=distinctive  AllPortsSameDT=off  OutDataTypeStr=boolean
  RX buffers : Subsystem  Priority=20
  Sum4 : Sum  Inputs=|++
  TX buffers CAN1 : Subsystem  Priority=20
  TX buffers CAN2 : Subsystem  Priority=20
  send_new_msg_CAN1 : Outport
  receive new msg CAN1 : Outport  Port=2
  send_new_msg_CAN2 : Outport  Port=3
  receive_new_msg_CAN2 : Outport  Port=4
  wires:
  basic_cycle_activation/1 -> Equal1/2
  new_message_CAN1/1 -> NOT/1
  current_basic_cycle/1 -> Equal1/1
  Constant21/1 -> Sum4/2
  Sum4/1 -> GreaterThan1/2
  Equal1/1 -> AND/1
  GreaterThan/1 -> AND/2
  GreaterThan1/1 -> AND/3
  AND5/1 -> TX buffers CAN1/Enable
  Constant22/1 -> Minus/2
  Minus/1 -> Mod/1
  Constant24/1 -> Mod/2
  Constant27/1 -> Mod1/2
  Minus1/1 -> Mod1/1
  Equal16/1 -> AND6/2
  AND6/1 -> RX buffers/Enable
  NOT3/1 -> AND7/1
  new_message_CAN2/1 -> NOT3/1
  Equal2/1 -> AND1/2
  Tx_condition/1 -> NOT2/1, NOT1/1, AND10/2, AND9/2, AND8/2, AND5/2
  AND1/1 -> AND4/1, AND7/2
  NOT/1 -> AND4/2
  AND4/1 -> receive new msg CAN1/1
  AND7/1 -> receive_new_msg_CAN2/1
  Constant16/1 -> Mod2/2
  Minus2/1 -> Mod2/1
  Constant10/1 -> Minus2/2
  AND8/1 -> TX buffers CAN2/Enable
  AND9/1 -> send_new_msg_CAN1/1
  AND10/1 -> send_new_msg_CAN2/1
  AND/1 -> AND8/1, AND9/1, AND10/1, AND5/1, AND1/1, AND6/1
  TM_COMM/1 -> Minus/3, Minus2/3, Minus4/2, Minus3/2, Minus1/2, Equal2/2, Equal16/2, Sum4/1, GreaterThan/2
  Minus3/1 -> Mod3/1
  Constant17/1 -> Mod3/2
  Data Store Read2/1 -> GreaterThan2/1
  Constant6/1 -> GreaterThan2/2
  Constant7/1 -> GreaterThan3/2
  Data Store Read3/1 -> GreaterThan3/1
  GreaterThan2/1 -> AND9/3, AND5/3
  GreaterThan3/1 -> AND10/3, AND8/3
  Equal4/1 -> AND5/4
  Mod/1 -> Equal4/1
  Constant8/1 -> Equal4/2
  Constant9/1 -> Equal6/2
  Mod2/1 -> Equal6/1
  Constant11/1 -> Equal7/2
  Constant12/1 -> Equal8/2
  Mod3/1 -> Equal8/1
  Mod1/1 -> Equal7/1
  Equal6/1 -> AND8/4
  Equal7/1 -> AND9/4
  Equal8/1 -> AND10/4
  Tx_ID/1 -> RX buffers/1(Rx_ID), TX buffers CAN1/1(Tx_ID), TX buffers CAN2/1(Tx_ID)
  NOT1/1 -> AND1/3
  Extra_Activation_Condition/1 -> AND/4
  Msg_Value_Data/1 -> TX buffers CAN2/2(Msg_Value_Data), TX buffers CAN1/2(Msg_Value_Data)
  local_time/1 -> GreaterThan1/1, Equal16/1, Equal2/1, Minus3/1, Minus1/1, Minus4/1, Minus2/1, Minus/1, GreaterThan/1
  NOT2/1 -> AND6/3
  Constant1/1 -> Equal/2
  Minus4/1 -> Equal/1
  Equal/1 -> AND10/5, AND9/5

== system HANcoder_E407_GTSync_v6/HANcoder STM32 Target - E407-STM32 algorithm/Global Ticks Increment/CAN Management/Matrix Cycle Manager/COMP Task - Check Timeouts ==
  note: BC 0 TW13
      | Timeout check
  basic cycle : Inport
  local time : Inport  Port=2
  AND : Logic  IconShape=distinctive  AllPortsSameDT=off  OutDataTypeStr=boolean
  Constant : Constant  Value=TM_Check_TOuts
  Constant5 : Constant  Value=0
  Equal : RelationalOperator  Operator===  OutDataTypeStr=boolean  RndMeth=Simplest
  Equal1 : RelationalOperator  Operator===  OutDataTypeStr=boolean  RndMeth=Simplest
  Timeout and Board error counter : Subsystem
  wires:
  Constant/1 -> Equal/2
  local time/1 -> Equal/1
  Constant5/1 -> Equal1/2
  basic cycle/1 -> Equal1/1
  Equal1/1 -> AND/1
  Equal/1 -> AND/2
  AND/1 -> Timeout and Board error counter/Enable

== system HANcoder_E407_GTSync_v6/HANcoder STM32 Target - E407-STM32 algorithm/Global Ticks Increment/CAN Management/Matrix Cycle Manager/COMP Task - New Master ==
  note: BC 0 TW14
      | New Master decision
  basic cycle : Inport
  local time : Inport  Port=2
  AND : Logic  IconShape=distinctive  AllPortsSameDT=off  OutDataTypeStr=boolean
  Constant : Constant  Value=TM_New_Master
  Constant5 : Constant  Value=0
  Equal : RelationalOperator  Operator===  OutDataTypeStr=boolean  RndMeth=Simplest
  Equal1 : RelationalOperator  Operator===  OutDataTypeStr=boolean  RndMeth=Simplest
  New Master : Subsystem
  wires:
  AND/1 -> New Master/Enable
  Equal/1 -> AND/2
  Equal1/1 -> AND/1
  basic cycle/1 -> Equal1/1
  Constant5/1 -> Equal1/2
  local time/1 -> Equal/1
  Constant/1 -> Equal/2

== system HANcoder_E407_GTSync_v6/HANcoder STM32 Target - E407-STM32 algorithm/Global Ticks Increment/CAN Management/Matrix Cycle Manager/COMP Task - Reset Board ==
  note: BC 0 TW16
      | Reset Board
  basic cycle : Inport
  local time : Inport  Port=2
  AND : Logic  Inputs=3  IconShape=distinctive  AllPortsSameDT=off  OutDataTypeStr=boolean
  Constant : Constant  Value=TM_Reset_Board
  Constant5 : Constant  Value=0
  Data Store Read : DataStoreRead  DataStoreName=Reset_Board
  Equal : RelationalOperator  Operator===  OutDataTypeStr=boolean  RndMeth=Simplest
  Equal1 : RelationalOperator  Operator===  OutDataTypeStr=boolean  RndMeth=Simplest
  RESET Board - Return to initialization : Subsystem  TreatAsAtomicUnit=on
  wires:
  AND/1 -> RESET Board - Return to initialization/Enable
  Equal/1 -> AND/2
  Equal1/1 -> AND/1
  basic cycle/1 -> Equal1/1
  Constant5/1 -> Equal1/2
  local time/1 -> Equal/1
  Constant/1 -> Equal/2
  Data Store Read/1 -> AND/3  "reset_s"

== system HANcoder_E407_GTSync_v6/HANcoder STM32 Target - E407-STM32 algorithm/Global Ticks Increment/CAN Management/Matrix Cycle Manager/COMP Task - Reset Variables BC0 ==
  note: BC 0 TW15
      | Reset variables
  basic cycle : Inport
  local time : Inport  Port=2
  AND : Logic  IconShape=distinctive  AllPortsSameDT=off  OutDataTypeStr=boolean
  Constant : Constant  Value=TM_Reset_Var
  Constant5 : Constant  Value=0
  Equal : RelationalOperator  Operator===  OutDataTypeStr=boolean  RndMeth=Simplest
  Equal1 : RelationalOperator  Operator===  OutDataTypeStr=boolean  RndMeth=Simplest
  Reset variables : Subsystem
  wires:
  Constant/1 -> Equal/2
  local time/1 -> Equal/1
  Constant5/1 -> Equal1/2
  basic cycle/1 -> Equal1/1
  Equal1/1 -> AND/1
  Equal/1 -> AND/2
  AND/1 -> Reset variables/Enable

== system HANcoder_E407_GTSync_v6/HANcoder STM32 Target - E407-STM32 algorithm/Global Ticks Increment/CAN Management/Matrix Cycle Manager/COMP Task - Reset Variables BC1 ==
  note: BC 1 TW17
      | Reset Variables
  basic cycle : Inport
  local time : Inport  Port=2
  AND : Logic  IconShape=distinctive  AllPortsSameDT=off  OutDataTypeStr=boolean
  Constant : Constant  Value=TM_Reset_Var
  Constant5 : Constant
  Equal : RelationalOperator  Operator===  OutDataTypeStr=boolean  RndMeth=Simplest
  Equal1 : RelationalOperator  Operator===  OutDataTypeStr=boolean  RndMeth=Simplest
  Reset Variables : Subsystem
  wires:
  AND/1 -> Reset Variables/Enable
  Equal/1 -> AND/2
  Equal1/1 -> AND/1
  basic cycle/1 -> Equal1/1
  Constant5/1 -> Equal1/2
  local time/1 -> Equal/1
  Constant/1 -> Equal/2

== system HANcoder_E407_GTSync_v6/HANcoder STM32 Target - E407-STM32 algorithm/Global Ticks Increment/CAN Management/Matrix Cycle Manager/COMP Task - Rx_Sync_bc0_Check ==
  note: Message information
  note: Reception condition
  note: Activation time conditions
  note: Activation extra condition:
      | LT not updated
  note: Transmision condition
  current_basic_cycle : Inport
  basic_cycle_activation : Inport  Port=2
  local_time : Inport  Port=3
  local_time_activation : Inport  Port=4
  Rx_condition : Inport  Port=5
  new_CAN1_msg : Inport  Port=6
  new_CAN2_msg : Inport  Port=7
  Rx_msg_CAN1 : Inport  Port=8  OutDataTypeStr=Bus: msg_buffer_type
  Rx_msg_CAN2 : Inport  Port=9  OutDataTypeStr=Bus: msg_buffer_type
  TM_COMM : Inport  Port=10
  Board_ID_Tx : Inport  Port=11
  Extra_activation_condition : Inport  Port=12
  AND : Logic  IconShape=distinctive  AllPortsSameDT=off  OutDataTypeStr=boolean
  AND1 : Logic  Inputs=3  IconShape=distinctive  AllPortsSameDT=off  OutDataTypeStr=boolean
  AND2 : Logic  IconShape=distinctive  AllPortsSameDT=off  OutDataTypeStr=boolean
  Equal : RelationalOperator  Operator===  OutDataTypeStr=boolean  RndMeth=Simplest
  Equal1 : RelationalOperator  Operator===  OutDataTypeStr=boolean  RndMeth=Simplest
  NOT : Logic  Operator=NOT  IconShape=distinctive  AllPortsSameDT=off  OutDataTypeStr=boolean
  Process_Messages : Subsystem  Priority=20
  Reset Tx msg counter : Subsystem  TreatAsAtomicUnit=on
  wires:
  new_CAN2_msg/1 -> Process_Messages/2(new_CAN2_msg)
  new_CAN1_msg/1 -> Process_Messages/1(new_CAN1_msg)
  current_basic_cycle/1 -> Process_Messages/5(expected_basic_cycle), Equal1/1
  local_time/1 -> Equal/1
  TM_COMM/1 -> Process_Messages/6(TM_COMM)
  basic_cycle_activation/1 -> Equal1/2
  AND/1 -> Process_Messages/Enable
  Rx_msg_CAN1/1 -> Process_Messages/3(Rx_msg_CAN1)
  Rx_msg_CAN2/1 -> Process_Messages/4(Rx_Msg_CAN2)
  Equal1/1 -> AND1/1
  Equal/1 -> AND1/2
  AND1/1 -> AND/1, AND2/1
  AND2/1 -> Reset Tx msg counter/Enable
  Board_ID_Tx/1 -> Process_Messages/7(expected_board_id)
  Extra_activation_condition/1 -> AND1/3
  Rx_condition/1 -> NOT/1, AND/2
  NOT/1 -> AND2/2
  local_time_activation/1 -> Equal/2

== system HANcoder_E407_GTSync_v6/HANcoder STM32 Target - E407-STM32 algorithm/Global Ticks Increment/CAN Management/Matrix Cycle Manager/COMP Task - Rx_Sync_bc1_Check ==
  note: Transmision condition
  note: Activation extra condition:
      | LT not updated
  note: Activation time conditions
  note: Reception condition
  note: Message information
  current_basic_cycle : Inport
  basic_cycle_activation : Inport  Port=2
  local_time : Inport  Port=3
  local_time_activating : Inport  Port=4
  Rx_condition : Inport  Port=5
  new_CAN1_msg : Inport  Port=6
  new_CAN2_msg : Inport  Port=7
  Rx_msg_CAN1 : Inport  Port=8  OutDataTypeStr=Bus: msg_buffer_type
  Rx_msg_CAN2 : Inport  Port=9  OutDataTypeStr=Bus: msg_buffer_type
  TM_COMM : Inport  Port=10
  Board_ID_Tx : Inport  Port=11
  Extra_activation_condition : Inport  Port=12
  AND : Logic  IconShape=distinctive  AllPortsSameDT=off  OutDataTypeStr=boolean
  AND1 : Logic  Inputs=3  IconShape=distinctive  AllPortsSameDT=off  OutDataTypeStr=boolean
  AND2 : Logic  IconShape=distinctive  AllPortsSameDT=off  OutDataTypeStr=boolean
  Equal : RelationalOperator  Operator===  OutDataTypeStr=boolean  RndMeth=Simplest
  Equal1 : RelationalOperator  Operator===  OutDataTypeStr=boolean  RndMeth=Simplest
  NOT : Logic  Operator=NOT  IconShape=distinctive  AllPortsSameDT=off  OutDataTypeStr=boolean
  Process_Messages : Subsystem  Priority=20
  Reset Tx msg counter : Subsystem  TreatAsAtomicUnit=on
  wires:
  NOT/1 -> AND2/2
  Rx_condition/1 -> AND/2, NOT/1
  Extra_activation_condition/1 -> AND1/3
  Board_ID_Tx/1 -> Process_Messages/7(expected_board_id)
  AND2/1 -> Reset Tx msg counter/Enable
  AND1/1 -> AND2/1, AND/1
  Equal/1 -> AND1/2
  Equal1/1 -> AND1/1
  Rx_msg_CAN2/1 -> Process_Messages/4(Rx_Msg_CAN2)
  Rx_msg_CAN1/1 -> Process_Messages/3(Rx_msg_CAN1)
  AND/1 -> Process_Messages/Enable
  basic_cycle_activation/1 -> Equal1/2
  TM_COMM/1 -> Process_Messages/6(TM_COMM)
  local_time/1 -> Equal/1
  current_basic_cycle/1 -> Equal1/1, Process_Messages/5(expected_basic_cycle)
  new_CAN1_msg/1 -> Process_Messages/1(new_CAN1_msg)
  new_CAN2_msg/1 -> Process_Messages/2(new_CAN2_msg)
  local_time_activating/1 -> Equal/2

== system HANcoder_E407_GTSync_v6/HANcoder STM32 Target - E407-STM32 algorithm/Global Ticks Increment/CAN Management/Matrix Cycle Manager/COMP Task - Rx_Vote1_Check ==
  note: Message information
  note: Reception condition
  note: Activation time conditions
  note: Activation extra condition:
      | LT not updated
  note: Transmision condition
  current_basic_cycle : Inport
  basic_cycle_activation : Inport  Port=2
  local_time : Inport  Port=3
  local_time_activation : Inport  Port=4
  Rx_condition : Inport  Port=5
  new_CAN1_msg : Inport  Port=6
  new_CAN2_msg : Inport  Port=7
  Rx_msg_CAN1 : Inport  Port=8  OutDataTypeStr=Bus: msg_buffer_type
  Rx_msg_CAN2 : Inport  Port=9  OutDataTypeStr=Bus: msg_buffer_type
  TM_COMM : Inport  Port=10
  Board_ID_Tx : Inport  Port=11
  Extra_activation_condition : Inport  Port=12
  AND : Logic  IconShape=distinctive  AllPortsSameDT=off  OutDataTypeStr=boolean
  AND1 : Logic  Inputs=3  IconShape=distinctive  AllPortsSameDT=off  OutDataTypeStr=boolean
  AND2 : Logic  IconShape=distinctive  AllPortsSameDT=off  OutDataTypeStr=boolean
  Equal : RelationalOperator  Operator===  OutDataTypeStr=boolean  RndMeth=Simplest
  Equal1 : RelationalOperator  Operator===  OutDataTypeStr=boolean  RndMeth=Simplest
  NOT : Logic  Operator=NOT  IconShape=distinctive  AllPortsSameDT=off  OutDataTypeStr=boolean
  Process_Messages : Subsystem  Priority=20
  Reset Tx msg counter : Subsystem  TreatAsAtomicUnit=on
  wires:
  new_CAN2_msg/1 -> Process_Messages/2(new_CAN2_msg)
  new_CAN1_msg/1 -> Process_Messages/1(new_CAN1_msg)
  current_basic_cycle/1 -> Equal1/1
  local_time/1 -> Equal/1
  TM_COMM/1 -> Process_Messages/5(TM_COMM)
  basic_cycle_activation/1 -> Equal1/2
  AND/1 -> Process_Messages/Enable
  Rx_msg_CAN1/1 -> Process_Messages/3(Rx_msg_CAN1)
  Rx_msg_CAN2/1 -> Process_Messages/4(Rx_Msg_CAN2)
  Equal1/1 -> AND1/1
  Equal/1 -> AND1/2
  AND1/1 -> AND/1, AND2/1
  AND2/1 -> Reset Tx msg counter/Enable
  Board_ID_Tx/1 -> Process_Messages/6(expected_board_id)
  Extra_activation_condition/1 -> AND1/3
  Rx_condition/1 -> NOT/1, AND/2
  NOT/1 -> AND2/2
  local_time_activation/1 -> Equal/2

== system HANcoder_E407_GTSync_v6/HANcoder STM32 Target - E407-STM32 algorithm/Global Ticks Increment/CAN Management/Matrix Cycle Manager/COMP Task - Rx_Vote2_Check ==
  note: Message information
  note: Reception condition
  note: Activation time conditions
  note: Activation extra condition:
      | LT not updated
  note: Transmision condition
  current_basic_cycle : Inport
  basic_cycle_activation : Inport  Port=2
  local_time : Inport  Port=3
  local_time_activating : Inport  Port=4
  Rx_condition : Inport  Port=5
  new_CAN1_msg : Inport  Port=6
  new_CAN2_msg : Inport  Port=7
  Rx_msg_CAN1 : Inport  Port=8  OutDataTypeStr=Bus: msg_buffer_type
  Rx_msg_CAN2 : Inport  Port=9  OutDataTypeStr=Bus: msg_buffer_type
  TM_COMM : Inport  Port=10
  Board_ID_Tx : Inport  Port=11
  Extra_activation_condition : Inport  Port=12
  AND : Logic  IconShape=distinctive  AllPortsSameDT=off  OutDataTypeStr=boolean
  AND1 : Logic  Inputs=3  IconShape=distinctive  AllPortsSameDT=off  OutDataTypeStr=boolean
  AND2 : Logic  IconShape=distinctive  AllPortsSameDT=off  OutDataTypeStr=boolean
  Equal : RelationalOperator  Operator===  OutDataTypeStr=boolean  RndMeth=Simplest
  Equal1 : RelationalOperator  Operator===  OutDataTypeStr=boolean  RndMeth=Simplest
  NOT : Logic  Operator=NOT  IconShape=distinctive  AllPortsSameDT=off  OutDataTypeStr=boolean
  Process_Messages : Subsystem  Priority=20
  Reset Tx msg counter : Subsystem  TreatAsAtomicUnit=on
  wires:
  new_CAN2_msg/1 -> Process_Messages/2(new_CAN2_msg)
  new_CAN1_msg/1 -> Process_Messages/1(new_CAN1_msg)
  current_basic_cycle/1 -> Equal1/1
  local_time/1 -> Equal/1
  TM_COMM/1 -> Process_Messages/5(TM_COMM)
  basic_cycle_activation/1 -> Equal1/2
  AND/1 -> Process_Messages/Enable
  Rx_msg_CAN1/1 -> Process_Messages/3(Rx_msg_CAN1)
  Rx_msg_CAN2/1 -> Process_Messages/4(Rx_Msg_CAN2)
  Equal1/1 -> AND1/1
  Equal/1 -> AND1/2
  AND1/1 -> AND/1, AND2/1
  AND2/1 -> Reset Tx msg counter/Enable
  Board_ID_Tx/1 -> Process_Messages/6(expected_board_id)
  Extra_activation_condition/1 -> AND1/3
  Rx_condition/1 -> NOT/1, AND/2
  NOT/1 -> AND2/2
  local_time_activating/1 -> Equal/2
